simulink model "enmod_nosie"  (R2021b)
settings: Solver=VariableStepAuto  StartTime=0.0  StopTime=3000  RelTol=1e-3
libraries: dsparch4 x2, dspmtrx3 x1, simulink x1, simulink_extras x1
settings Model: Creator=lucas  LastModifiedBy=lucas

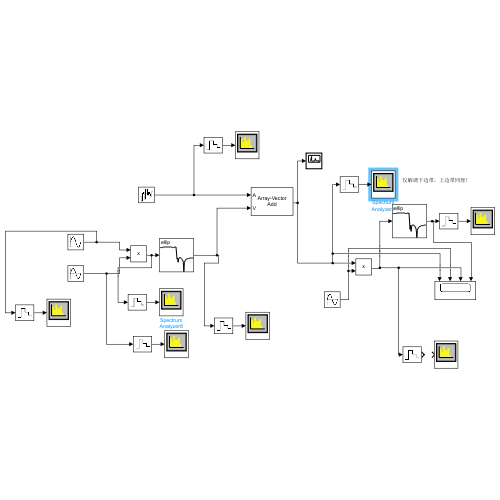
[thumbnail: Simulink's stored preview of the top-level diagram]
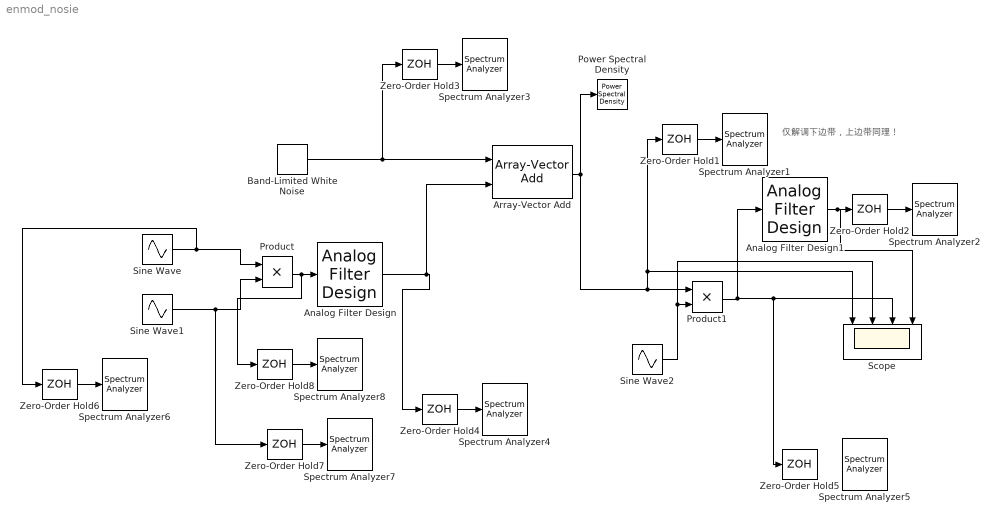
== system enmod_nosie ==
  note: 仅解调下边带，上边带同理！
  Analog Filter Design : dsparch4/Analog Filter Design  method=Elliptic  filttype=Lowpass  N=8  Wlo=2*pi*18  Whi=80  Rp=2  Rs=40
  Analog Filter Design1 : dsparch4/Analog Filter Design  method=Elliptic  filttype=Lowpass  N=10  Wlo=4*pi  Whi=80  Rp=2  Rs=40
  Array-Vector Add : dspmtrx3/Array-Vector Add  Dimension=1  V_Source=Input port  V_VectFromMask=[0.5 0.25]  prodOutputSignedness=Auto  roundingMode=Floor  overflowMode=off  firstCoeffSignedness=Auto  firstCoeffDataTypeStr=Inherit: Same word length as input  firstCoeffMin=[]  firstCoeffMax=[]  firstCoeffLastDataTypeStr=Inherit: Same word length as input  accumSignedness=Auto  outputSignedness=Auto  outputDataTypeStr=Inherit: Same as accumulator  outputMin=[]  outputMax=[]  outputLastDataTypeStr=Inherit: Same as accumulator
      settings: SourceProductBaseCode=DS
  Band-Limited White Noise : simulink/Sources/Band-Limited White Noise  Cov=1  Ts=0.1  seed=[23341]
  Power Spectral Density : simulink_extras/Additional Sinks/Power Spectral Density  npts=128  fftpts=512  HowOften=64  sampleT=0.1
      settings: SourceProductBaseCode=SL
  Product : Product
  Product1 : Product
  Scope : Scope  NumInputPorts=4
  Sine Wave : Sin  Amplitude=2  Frequency=2*pi*2  SampleTime=0
  Sine Wave1 : Sin  Amplitude=2  Frequency=125.664  SampleTime=0
  Sine Wave2 : Sin  Amplitude=2  Frequency=2*pi*20  SampleTime=0
  Spectrum Analyzer{1..8} (8 alike) : SpectrumAnalyzer
  Zero-Order Hold{1..8} (8 alike) : ZeroOrderHold  SampleTime=-1
  wires:
  Analog Filter Design/1 -> Array-Vector Add/2, Zero-Order Hold4/1
  Zero-Order Hold4/1 -> Spectrum Analyzer4/1
  Sine Wave/1 -> Product/1, Zero-Order Hold6/1
  Zero-Order Hold6/1 -> Spectrum Analyzer6/1
  Sine Wave1/1 -> Zero-Order Hold7/1, Product/2
  Zero-Order Hold7/1 -> Spectrum Analyzer7/1
  Product/1 -> Zero-Order Hold8/1, Analog Filter Design/1
  Zero-Order Hold8/1 -> Spectrum Analyzer8/1
  Zero-Order Hold3/1 -> Spectrum Analyzer3/1
  Band-Limited White Noise/1 -> Zero-Order Hold3/1, Array-Vector Add/1
  Zero-Order Hold2/1 -> Spectrum Analyzer2/1
  Product1/1 -> Analog Filter Design1/1, Zero-Order Hold5/1, Scope/3
  Zero-Order Hold1/1 -> Spectrum Analyzer1/1
  Array-Vector Add/1 -> Power Spectral Density/1, Zero-Order Hold1/1, Scope/1, Product1/1
  Sine Wave2/1 -> Scope/2, Product1/2
  Analog Filter Design1/1 -> Scope/4, Zero-Order Hold2/1
